simulink model "softMBD"  (R2025b)
settings: Solver=FixedStepAuto  StartTime=0.0  StopTime=30  FixedStep=0.005  RelTol=1e-3
values from neighbouring files (symbols this model uses):
  FPV_mass = 0.8    [Soft.m]
  g = 9.81    [Soft.m]
  ks = 0    [Soft.m]
  p_0 = 1013.25    [Soft.m]
  Q2Ts = forcetomotors()    [Soft.m]    (also in forcetomotors.m = inv(Ts2Q))
  takeOffDuration = 2    [Soft.m]
  Ts = 0.005    [Soft.m]
undefined symbols (not defined in the file or in its folder): CdA, DiscIntNeverNeededParam, kd_pq, kd_pr, kd_y, ki_pq, ki_pr, ki_y, kp_pq, kp_pr, kp_y, pInitialization, rho
libraries: simulink x37, discretizing x11, slpidlib x2, SignalEditorBlockLib x1, simulink_extras x1, shared6dof x1, dynamicsLibrary x1, aerolibasang x1, aerolibnav x1
(part 1 of 20)
settings Model: Creator=rafal  LastModifiedBy=rafal
settings DataIOCC: ReturnWorkspaceOutputs=off
settings OptimizationCC: DefaultParameterBehavior=Inlined  UseDivisionForNetSlopeComputation=on  GainParamInheritBuiltInType=on  UseFloatMulNetSlope=on  InlineInvariantSignals=on  PassReuseOutputArgsAs=Individual arguments  ZeroExternalMemoryAtStartup=off  ZeroInternalMemoryAtStartup=off  NoFixptDivByZeroProtection=on  EfficientFloat2IntCast=on  LifeSpan=1  OptimizeBlockOrder=speed  DifferentSizesBufferReuse=on  EfficientTunableParamExpr=on
settings DebuggingCC: ParameterTunabilityLossMsg=error  BusObjectLabelMismatch=error
settings HardwareCC: ProdBitPerPointer=32.0  ProdBitPerSizeT=32.0  ProdBitPerPtrDiffT=32.0  ProdLargestAtomicInteger=Long  ProdLargestAtomicFloat=Double  ProdWordSize=32.0  ProdLongLongMode=on  ProdHWDeviceType=ARM Compatible->ARM Cortex-M
settings SFSimCC: MATLABDynamicMemAlloc=off
settings RTWCC: SystemTargetFile=ert.tlc  GenCodeOnly=on  TemplateMakefile=ert_default_tmf  Description=Embedded Coder
settings CodeAppCC: ForceParamTrailComments=on  IgnoreCustomStorageClasses=off  OperatorAnnotations=on  SimulinkDataObjDesc=on  SFDataObjDesc=on  CustomSymbolStrGlobalVar=rt$N$M  CustomSymbolStrType=$N$M  CustomSymbolStrFcn=$N$M$F  CustomSymbolStrMacro=$N$M  InsertBlockDesc=on
settings ERTTargetCC: ERTCustomFileTemplate=example_file_process.tlc  ERTFilePackagingFormat=CompactWithDataFile  TargetLangStandard=C99 (ISO)  IncludeMdlTerminateFcn=off  CombineSignalStateStructs=on  SupportContinuousTime=on  SupportNonInlinedSFcns=on

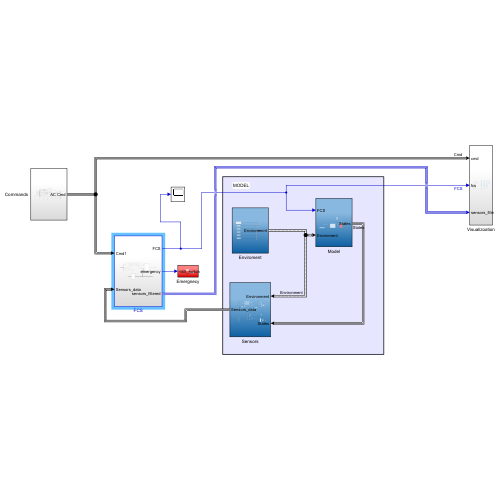
[thumbnail: Simulink's stored preview of the top-level diagram]
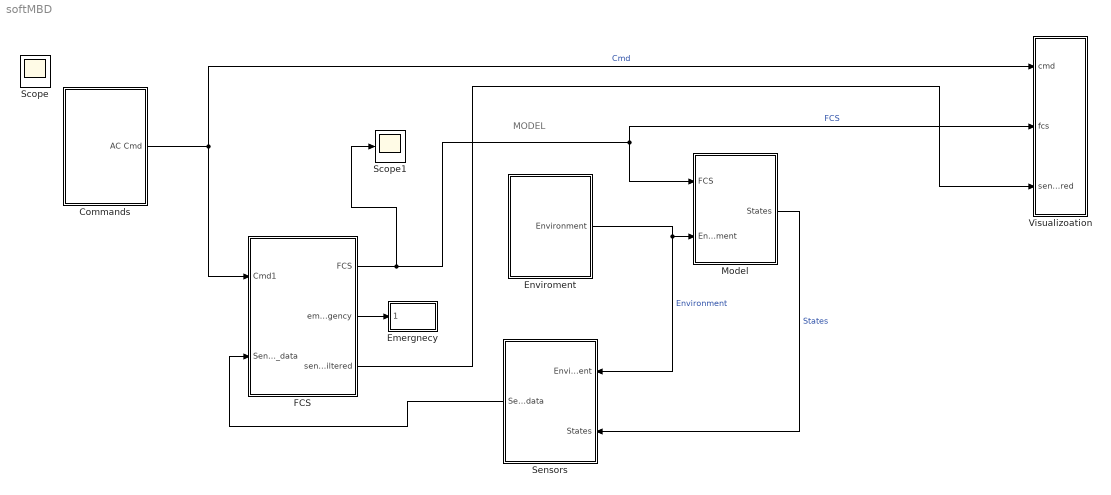
== system softMBD ==
  note: MODEL
  Commands : Subsystem
  Emergnecy : Subsystem
  Enviroment : Subsystem
  FCS : Subsystem
  Model : Subsystem
  Scope1 : Scope
      settings: ActiveDisplayYMinimum=-145.65311813354487  ActiveDisplayYMaximum=2290.6281242370605
  Sensors : Subsystem
  Visualizoation : Subsystem
  Scope : Scope
  wires:
  Model/1(States) -> Sensors/2(States)  "States"
  Sensors/1(Sensors_data) -> FCS/2(Sensors_data)
  Commands/1(AC Cmd) -> Visualizoation/1(cmd), FCS/1(Cmd1)  "Cmd"
  FCS/1(FCS) -> Scope1/1, Visualizoation/2(fcs), Model/1(FCS)  "FCS"
  FCS/2(emergency) -> Emergnecy/1(<kill_switch>)
  Enviroment/1(Environment) -> Sensors/1(Environment), Model/2(Enviroment)  "Environment"
  FCS/3(sensors_filtered) -> Visualizoation/3(sensors_filtered)

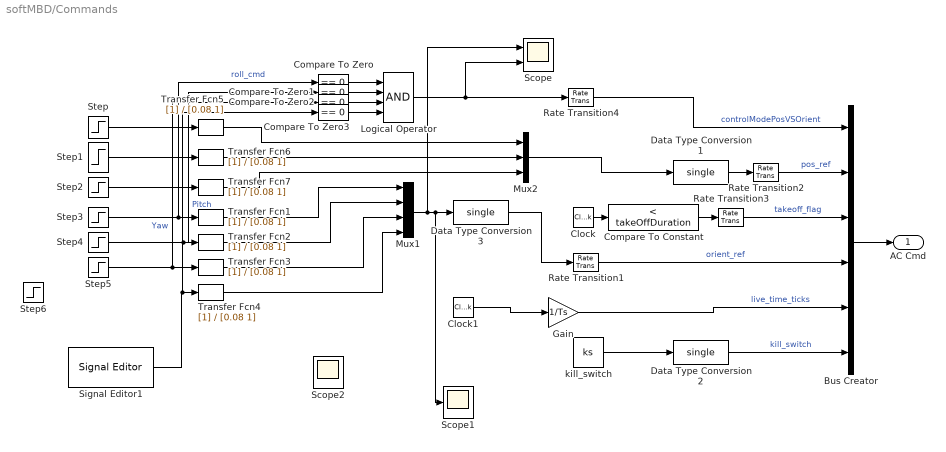
== system softMBD/Commands ==
  Bus Creator : BusCreator  Inputs=6  OutDataTypeStr=Bus: CommandBus
  Clock : DigitalClock  SampleTime=0.005
  Clock1 : DigitalClock  SampleTime=0.005
  Compare To Constant : simulink/Logic and Bit Operations/Compare To Constant  relop=<  const=takeOffDuration  OutDataTypeStr=boolean
  Compare To Zero : simulink/Logic and Bit Operations/Compare To Zero  relop===  OutDataTypeStr=uint8
  Compare To Zero1 : simulink/Logic and Bit Operations/Compare To Zero  relop===  OutDataTypeStr=uint8
  Compare To Zero2 : simulink/Logic and Bit Operations/Compare To Zero  relop===  OutDataTypeStr=boolean
  Compare To Zero3 : simulink/Logic and Bit Operations/Compare To Zero  relop===  OutDataTypeStr=boolean
  Data Type Conversion1 : DataTypeConversion  OutDataTypeStr=single  SaturateOnIntegerOverflow=off  RndMeth=Floor
  Data Type Conversion2 : DataTypeConversion  OutDataTypeStr=single  SaturateOnIntegerOverflow=off  RndMeth=Floor
  Data Type Conversion3 : DataTypeConversion  OutDataTypeStr=single  SaturateOnIntegerOverflow=off  RndMeth=Floor
  Gain : Gain  Gain=1/Ts  OutDataTypeStr=single
  Logical Operator : Logic  Inputs=4  AllPortsSameDT=off  OutDataTypeStr=boolean
  Mux1 : Mux
  Mux2 : Mux  Inputs=3
  Rate Transition{1..4} (4 alike) : RateTransition  OutPortSampleTime=Ts
  Scope : Scope  NumInputPorts=2
      settings: ActiveDisplayYMinimum=-0.12499999999999997  ActiveDisplayYMaximum=1.125  DataLoggingVariableName=ScopeData74
  Scope1 : Scope
      settings: ActiveDisplayYMinimum=-1  ActiveDisplayYMaximum=1  DataLoggingVariableName=ScopeData25
  Scope2 : Scope
      settings: ActiveDisplayYMinimum=-0.11809653934888488  ActiveDisplayYMaximum=1.0178996154832094  DataLoggingVariableName=ScopeData40
  Signal Editor1 : SignalEditorBlockLib/Signal Editor  FileName=signal-test.mat  ActiveScenario=Scenario  ActiveSignal=Signal 1  IsBus=off  OutputBusObjectStr=Bus: BusObject  SampleTime=0  ZeroCross=off  OutputAfterFinalValue=Setting to zero  Unit=inherit  PreserveSignalName=on  ApplySigPropsToAllScenarios=on  ApplySigPropsToAllSignals=off  SignalPropertySource=Dialog parameters
  Step{,1..5} (6 alike) : Step  After=0  SampleTime=0
  Step6 : Step  Time=2  Before=1  After=0  SampleTime=0
  Transfer Fcn{1..7} (7 alike) : TransferFcn  Denominator=[0.08 1]
  kill_switch : Constant  Value=ks
  AC Cmd : Outport  OutDataTypeStr=Bus: CommandBus  VectorParamsAs1DForOutWhenUnconnected=off
  wires:
  Rate Transition4/1 -> Bus Creator/1  "controlModePosVSOrient"
  Gain/1 -> Bus Creator/5  "live_time_ticks"
  Clock/1 -> Compare To Constant/1
  Step1/1 -> Transfer Fcn6/1
  Rate Transition2/1 -> Bus Creator/2  "pos_ref"
  Step2/1 -> Transfer Fcn7/1
  Mux1/1 -> Scope/1, Scope1/1, Data Type Conversion3/1
  Bus Creator/1 -> AC Cmd/1
  Compare To Constant/1 -> Rate Transition3/1
  Step4/1 -> Compare To Zero1/1, Transfer Fcn2/1  "Pitch"
  Data Type Conversion1/1 -> Rate Transition2/1
  Data Type Conversion3/1 -> Rate Transition1/1
  Step/1 -> Transfer Fcn5/1
  Mux2/1 -> Data Type Conversion1/1
  Rate Transition1/1 -> Bus Creator/4  "orient_ref"
  Step5/1 -> Compare To Zero2/1, Transfer Fcn3/1  "Yaw"
  Rate Transition3/1 -> Bus Creator/3  "takeoff_flag"
  Compare To Zero/1 -> Logical Operator/1
  Compare To Zero1/1 -> Logical Operator/2
  Compare To Zero2/1 -> Logical Operator/3
  kill_switch/1 -> Data Type Conversion2/1
  Data Type Conversion2/1 -> Bus Creator/6  "kill_switch"
  Clock1/1 -> Gain/1
  Step3/1 -> Compare To Zero/1, Transfer Fcn1/1  "roll_cmd"
  Transfer Fcn1/1 -> Mux1/1
  Transfer Fcn3/1 -> Mux1/3
  Transfer Fcn4/1 -> Mux1/4
  Transfer Fcn5/1 -> Mux2/1
  Transfer Fcn6/1 -> Mux2/2
  Transfer Fcn7/1 -> Mux2/3
  Compare To Zero3/1 -> Logical Operator/4
  Transfer Fcn2/1 -> Mux1/2
  Logical Operator/1 -> Rate Transition4/1, Scope/2
  Signal Editor1/1 -> Compare To Zero3/1, Transfer Fcn4/1

== system softMBD/Emergnecy ==
  <kill_switch> : Inport
  If : If
  Switch Case Action Subsystem : Subsystem  TreatAsAtomicUnit=on
  Terminator : Terminator
  Zero : Constant  OutDataTypeStr=Inherit: Inherit via back propagation
  wires:
  If/1 -> Switch Case Action Subsystem/Action
  If/2 -> Terminator/1
  Switch Case Action Subsystem/1(emergency) -> ?
  Zero/1 -> Switch Case Action Subsystem/1(In1)
  <kill_switch>/1 -> If/1

== system softMBD/Enviroment ==
  Air Density : Constant  Value=1.225  OutDataTypeStr=single
  Air Temp : Constant  Value=288  OutDataTypeStr=single
  Bus Creator : BusCreator  Inputs=6  OutDataTypeStr=Bus: AtmosphereBus  NonVirtualBus=on
  Gravity : Constant  Value=[0 0 9.81]  OutDataTypeStr=single
  Magnetic Field : Constant  Value=[0 0 0]  OutDataTypeStr=single
  Pressure : Constant  Value=1013.25  OutDataTypeStr=single
  Speed of Sound : Constant  Value=340  OutDataTypeStr=single
  Environment : Outport  VectorParamsAs1DForOutWhenUnconnected=off
  wires:
  Magnetic Field/1 -> Bus Creator/6  "MagneticField_ned"
  Air Density/1 -> Bus Creator/5  "air_density"
  Air Temp/1 -> Bus Creator/2  "air_temp"
  Gravity/1 -> Bus Creator/1  "Gravity_ned"
  Speed of Sound/1 -> Bus Creator/3  "speed_sound"
  Bus Creator/1 -> Environment/1
  Pressure/1 -> Bus Creator/4  "pressure"

== system softMBD/FCS ==
  Cmd1 : Inport
  Sensors_data : Inport  Port=2
  Bus Selector : BusSelector  OutputSignals=controlModePosVSOrient,orient_ref,takeoff_flag,pos_ref,kill_switch
  Controller : Subsystem
  filters : Subsystem
  value scaling : Subsystem
  FCS : Outport
  emergency : Outport  Port=2
  sensors_filtered : Outport  Port=3
  wires:
  Cmd1/1 -> Bus Selector/1
  Controller/1(FCS) -> FCS/1
  Bus Selector/1 -> Controller/1(In1)  "<controlModePosVSOrient>"
  Bus Selector/3 -> Controller/3(In3)  "<takeoff_flag>"
  Bus Selector/4 -> Controller/4(In4)  "<pos_ref>"
  Sensors_data/1 -> filters/1(Sensors_data)
  filters/1(Sensors_filtered) -> sensors_filtered/1, Controller/5(Sensors_filtered)  "sensors_filtered"
  Bus Selector/5 -> emergency/1  "<kill_switch>"
  Bus Selector/2 -> value scaling/1(<orient_ref>)  "<orient_ref>"
  value scaling/1(Out1) -> Controller/2(In2)

== system softMBD/Model ==
  FCS : Inport
  Enviroment : Inport  Port=2
  6DOF (Quaternion)1 : shared6dof/6DOF (Euler Angles)  units=Metric (MKS)  mtype=Fixed  rep=Euler Angles  xme_0=[0 0 0]  Vm_0=[0 0 0]  eul_0=[0 0 0]  pm_0=[0 0 0]  mass_0=FPV_mass  mass_e=0.5  mass_f=2.0  inertia=diag([0.003, 0.003, 0.005])  inertia_e=eye(3)  inertia_f=2*eye(3)  k_quat=Vehicle.SixDOF.quatGain  vre_flag=on  abi_flag=on  aMode=aMode  xme_statename=''  Vm_statename=''  eul_statename=''  quat_statename=''  pm_statename=''  mass_statename=''
  Abs : Abs  SaturateOnIntegerOverflow=off
  Add : Sum  Inputs=+++
  Bias : Bias  Bias=-48  SaturateOnIntegerOverflow=off
  Bias1 : Bias  Bias=200  SaturateOnIntegerOverflow=off
  Bus Creator : BusCreator  Inputs=8
  Bus Selector : BusSelector  OutputSignals=air_density
  Constant : Constant  Value=630*[1 1 1 1]  VectorParams1D=off
  Constant2 : Constant  Value=FPV_mass*g*[0 0 1]
  Data Type Conversion2 : DataTypeConversion  OutDataTypeStr=double  SaturateOnIntegerOverflow=off  RndMeth=Floor
  Data Type Conversion3 : DataTypeConversion  OutDataTypeStr=double  SaturateOnIntegerOverflow=off  RndMeth=Floor
  Gain : Gain  Commented=on  Gain=[1; 1; -1]
  Gain1 : Gain  Gain=(4184-200)/1999
  Gain2 : Gain  Gain=[1 -1 -1 1]
  Gain3 : Gain  Gain=-1/2*rho*CdA
  Matrix Multiply : Product  Multiplication=Matrix(*)
  Multirotor : Multirotor  armLength=0.11  radius=0.0635
  Product : Product
  Saturation : Saturate  UpperLimit=4184  LowerLimit=200
  Scope1 : Scope  NumInputPorts=3
      settings: ActiveDisplayYMinimum=-17.244801664132787  ActiveDisplayYMaximum=11.437507576273727  DataLoggingVariableName=ScopeData54
  Scope2 : Scope  NumInputPorts=2
      settings: ActiveDisplayYMinimum=-2865.3748027143724  ActiveDisplayYMaximum=2716.5327218117013  DataLoggingVariableName=ScopeData62
  Scope3 : Scope  NumInputPorts=4
      settings: ActiveDisplayYMinimum=-27.905959147776141  ActiveDisplayYMaximum=16.159289367560238  DataLoggingVariableName=ScopeData64
  Scope4 : Scope  NumInputPorts=2
      settings: ActiveDisplayYMinimum=-1  ActiveDisplayYMaximum=1  DataLoggingVariableName=ScopeData38
  Subsystem : Subsystem  Commented=on
  Terminator : Terminator
  States : Outport
  wires:
  6DOF (Quaternion)1/1 -> Scope3/1, Bus Creator/1  "V_e"
  6DOF (Quaternion)1/2 -> Scope3/4, Bus Creator/2  "x_e"
  6DOF (Quaternion)1/3 -> Bus Creator/3  "Euler"
  Bus Creator/1 -> States/1
  6DOF (Quaternion)1/4 -> Bus Creator/4  "DCM_be"
  6DOF (Quaternion)1/5 -> Abs/1, Bus Creator/5, Gain3/1  "V_b"
  6DOF (Quaternion)1/6 -> Scope3/3, Bus Creator/6  "omega_b"
  6DOF (Quaternion)1/7 -> Bus Creator/7  "Domega_b"
  6DOF (Quaternion)1/8 -> Scope3/2, Bus Creator/8  "Accel_b"
  Subsystem/1(F_xyz) -> Gain/1
  Bias/1 -> Gain1/1
  Saturation/1 -> Gain2/1
  Constant2/1 -> Add/2
  Enviroment/1 -> Bus Selector/1
  Data Type Conversion2/1 -> Multirotor/2
  Multirotor/1 -> Scope1/1, Add/3
  Bias1/1 -> Saturation/1
  Multirotor/2 -> Scope4/1, 6DOF (Quaternion)1/2
  FCS/1 -> Scope2/1, Data Type Conversion3/1
  Bus Selector/1 -> Data Type Conversion2/1  "<air_density>"
  Gain1/1 -> Bias1/1
  Data Type Conversion3/1 -> Bias/1
  Add/1 -> 6DOF (Quaternion)1/1, Scope1/2
  6DOF (Quaternion)1/9 -> Terminator/1  "Accel_b"
  Gain2/1 -> Scope2/2, Multirotor/1
  Gain3/1 -> Product/2
  Abs/1 -> Product/1
  Product/1 -> Add/1, Scope1/3

== system softMBD/Sensors ==
  note: altitude_sonar
  Environment : Inport
  States : Inport  Port=2
  Assumes takeoff was level1 : Bias  Commented=on  Bias=p_0  SaturateOnIntegerOverflow=off
  Bus Selector : BusSelector  Commented=on  OutputSignals=Accel_b,omega_b,Domega_b,DCM_be,x_e
  Bus Selector1 : BusSelector  Commented=on  OutputSignals=Gravity_ned
  Bus Selector2 : BusSelector  OutputSignals=x_e,V_e,omega_b,Accel_b
  CG location : Constant  Commented=on  Value=[0 0 0]
  Data Type Conversion1 : DataTypeConversion  Commented=on  OutDataTypeStr=single  SaturateOnIntegerOverflow=off  RndMeth=Floor
  Data Type Conversion2 : DataTypeConversion  Commented=on  OutDataTypeStr=single  SaturateOnIntegerOverflow=off  RndMeth=Floor
  Data Type Conversion3 : DataTypeConversion  Commented=on  OutDataTypeStr=single  SaturateOnIntegerOverflow=off  RndMeth=Floor
  Demux : Demux  Commented=on  Outputs=3
  Demux1 : Demux  Commented=on  Outputs=3
  Demux2 : Demux  Outputs=3
  Demux3 : Demux  Outputs=3
  Matrix Multiply : Product  Commented=on  Multiplication=Matrix(*)
  Memory : Memory  Commented=on
  Mux : Mux  Commented=on  Inputs=8
  Mux2 : Mux  Inputs=3
  Rate Transition : RateTransition  Commented=on
  Rate Transition1 : RateTransition
  Saturation : Saturate  Commented=on  UpperLimit=inf  LowerLimit=0  OutDataTypeStr=single
  Scope : Scope  Commented=on  NumInputPorts=3
      settings: ActiveDisplayYMinimum=-74.251567840576172  ActiveDisplayYMaximum=64.477069854736328  DataLoggingVariableName=ScopeData44
  Scope1 : Scope  Commented=on  NumInputPorts=3
      settings: ActiveDisplayYMinimum=-0.22507907450199127  ActiveDisplayYMaximum=0.16993089020252228  DataLoggingVariableName=ScopeData48
  Scope2 : Scope  Commented=on
      settings: ActiveDisplayYMinimum=-1  ActiveDisplayYMaximum=1  DataLoggingVariableName=ScopeData65
  Scope3 : Scope
      settings: ActiveDisplayYMinimum=-1  ActiveDisplayYMaximum=1  DataLoggingVariableName=ScopeData63
  Selector : Selector  Commented=on  InputPortWidth=3  IndexOptions=Index vector (dialog)  Indices=[3]  OutputSizes=1
  Subsystem : Subsystem  Commented=on
  Subsystem1 : Subsystem
  Terminator1 : Terminator
  Terminator2 : Terminator
  Terminator3 : Terminator
  Three-axis Inertial Measurement Unit1 : aerolibnav/Three-axis Inertial Measurement Unit  Commented=on  units=Metric (MKS)  imu=[0 0 0]  i_Ts=0  dtype_a=on  w_a=190  z_a=0.707  a_sf_cc=[1 0 0; 0 1 0; 0 0 1]  a_bias=[0 0 0]  a_sat="[-inf  -inf  -inf  inf inf inf]"  dtype_g=on  w_g=190  z_g=0.707  g_sf_cc=[1 0 0; 0 1 0; 0 0 1]  g_bias=[0 0 0]  g_sens=[0 0 0]  g_sat="[-inf  -inf  -inf  inf inf inf]"  i_rand=on  i_seeds=[23093 23094 23095 23096 23097 23098]  i_pow=[0.001 0.001 0.001 0.0001 0.0001 0.0001]
  altToprs_gain : Gain  Commented=on  Gain=12.017  ParamDataTypeStr=single  OutDataTypeStr=single
  altToprs_gain1 : Gain  Commented=on  Gain=-1  ParamDataTypeStr=single  OutDataTypeStr=double
  altToprs_gain2 : Gain  Gain=-1  ParamDataTypeStr=single  OutDataTypeStr=double
  altToprs_gain3 : Gain  Gain=-1  ParamDataTypeStr=single  OutDataTypeStr=double
  Sensors_data : Outport
  wires:
  Memory/1 -> Bus Selector/1
  Environment/1 -> Bus Selector1/1
  Bus Selector1/1 -> Matrix Multiply/2  "<Gravity_ned>"
  Bus Selector/4 -> Matrix Multiply/1  "<DCM_be>"
  CG location/1 -> Three-axis Inertial Measurement Unit1/4
  Matrix Multiply/1 -> Scope2/1, Three-axis Inertial Measurement Unit1/5
  Bus Selector/5 -> Selector/1  "<x_e>"
  Bus Selector/3 -> Three-axis Inertial Measurement Unit1/3  "<Domega_b>"
  Bus Selector/2 -> Three-axis Inertial Measurement Unit1/2  "<omega_b>"
  Bus Selector/1 -> Three-axis Inertial Measurement Unit1/1  "<Accel_b>"
  Selector/1 -> altToprs_gain/1, altToprs_gain1/1
  Saturation/1 -> Mux/8  "prs"
  Demux/1 -> Mux/1, Scope/1  "ddx"
  Demux/2 -> Mux/2, Scope/2  "ddy"
  Demux/3 -> Mux/3, Scope/3  "ddz"
  Demux1/1 -> Scope1/1, Mux/4  "p"
  Demux1/2 -> Scope1/2, Mux/5  "q"
  Demux1/3 -> Scope1/3, Mux/6  "r"
  Subsystem/1(Out1) -> Rate Transition/1
  altToprs_gain1/1 -> Saturation/1
  altToprs_gain/1 -> Assumes takeoff was level1/1
  Assumes takeoff was level1/1 -> Data Type Conversion2/1
  Three-axis Inertial Measurement Unit1/1 -> Data Type Conversion3/1  "prs"
  Data Type Conversion3/1 -> Demux/1
  Three-axis Inertial Measurement Unit1/2 -> Data Type Conversion1/1  "prs"
  Data Type Conversion1/1 -> Demux1/1
  Data Type Conversion2/1 -> Mux/7
  Demux2/3 -> altToprs_gain2/1
  Demux3/2 -> Mux2/2
  Rate Transition1/1 -> Sensors_data/1
  Demux3/1 -> Mux2/1
  Demux2/2 -> Terminator1/1
  Bus Selector2/1 -> Demux2/1  "<x_e>"
  altToprs_gain2/1 -> Scope3/1, Subsystem1/1(In1)
  Demux3/3 -> altToprs_gain3/1
  altToprs_gain3/1 -> Mux2/3
  States/1 -> Bus Selector2/1
  Mux2/1 -> Terminator3/1
  Subsystem1/1(Out1) -> Rate Transition1/1
  Demux2/1 -> Terminator2/1
  Bus Selector2/2 -> Demux3/1  "<V_e>"
  Bus Selector2/3 -> Subsystem1/2(In2)  "<omega_b>"
  Bus Selector2/4 -> Subsystem1/3(<Accel_b>)  "<Accel_b>"
  Mux/1 -> Subsystem/1(In1)

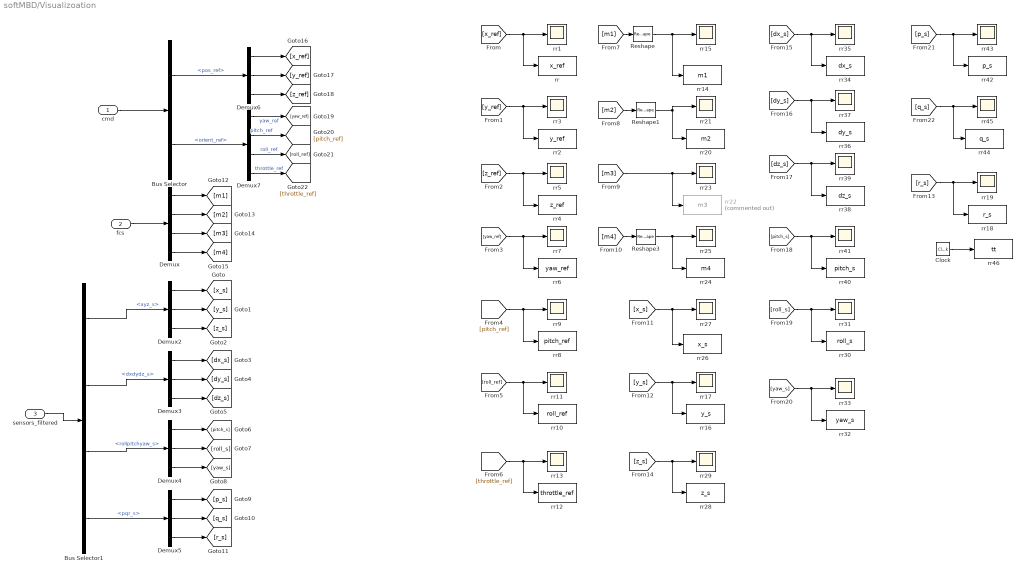
== system softMBD/Visualizoation ==
  cmd : Inport
  fcs : Inport  Port=2
  sensors_filtered : Inport  Port=3
  Bus Selector : BusSelector  OutputSignals=pos_ref,orient_ref
  Bus Selector1 : BusSelector  OutputSignals=xyz_s,dxdydz_s,rollpitchyaw_s,pqr_s
  Clock : DigitalClock  SampleTime=0.005
  Demux : Demux
  Demux{2..6} (5 alike) : Demux  Outputs=3
  Demux7 : Demux
  Reshape : Reshape
  Reshape1 : Reshape
  Reshape3 : Reshape
  rr : ToWorkspace  VariableName=x_ref  SampleTime=Ts
  rr{1,3,5,7,9,11,13,15,17,19,21,23,25,27,29,31,33,35,37,39,41,43,45} (23 alike) : Scope
      rr1 settings: ActiveDisplayYMinimum=-1  ActiveDisplayYMaximum=1  DataLoggingVariableName=ScopeData10
      rr11 settings: ActiveDisplayYMinimum=-1  ActiveDisplayYMaximum=1  DataLoggingVariableName=ScopeData6
      rr13 settings: ActiveDisplayYMinimum=-1  ActiveDisplayYMaximum=1  DataLoggingVariableName=ScopeData7
      rr15 settings: ActiveDisplayYMinimum=-73.950467746195855  ActiveDisplayYMaximum=1145.5542097157629  DataLoggingVariableName=ScopeData8
      rr17 settings: ActiveDisplayYMinimum=-1  ActiveDisplayYMaximum=1  DataLoggingVariableName=ScopeData9
      rr19 settings: ActiveDisplayYMinimum=-1  ActiveDisplayYMaximum=1  DataLoggingVariableName=ScopeData11
      rr21 settings: ActiveDisplayYMinimum=38  ActiveDisplayYMaximum=58  DataLoggingVariableName=ScopeData12
      rr23 settings: ActiveDisplayYMinimum=-70.597177763307627  ActiveDisplayYMaximum=1115.3745998697689  DataLoggingVariableName=ScopeData13
      rr25 settings: ActiveDisplayYMinimum=46.949385488802776  ActiveDisplayYMaximum=57.45553060077502  DataLoggingVariableName=ScopeData14
      rr27 settings: ActiveDisplayYMinimum=-1  ActiveDisplayYMaximum=1  DataLoggingVariableName=ScopeData15
      rr29 settings: ActiveDisplayYMinimum=-248.57406984307249  ActiveDisplayYMaximum=124.72069577188705  DataLoggingVariableName=ScopeData16
      rr3 settings: ActiveDisplayYMinimum=-5  ActiveDisplayYMaximum=5  DataLoggingVariableName=ScopeData2
      rr31 settings: ActiveDisplayYMinimum=-1  ActiveDisplayYMaximum=1  DataLoggingVariableName=ScopeData17
      rr33 settings: ActiveDisplayYMinimum=-1  ActiveDisplayYMaximum=1  DataLoggingVariableName=ScopeData18
      rr35 settings: ActiveDisplayYMinimum=-1  ActiveDisplayYMaximum=1  DataLoggingVariableName=ScopeData19
      rr37 settings: ActiveDisplayYMinimum=-1  ActiveDisplayYMaximum=1  DataLoggingVariableName=ScopeData20
      rr39 settings: ActiveDisplayYMinimum=-1  ActiveDisplayYMaximum=1  DataLoggingVariableName=ScopeData21
      rr41 settings: ActiveDisplayYMinimum=-1  ActiveDisplayYMaximum=1  DataLoggingVariableName=ScopeData22
      rr43 settings: ActiveDisplayYMinimum=-1  ActiveDisplayYMaximum=1  DataLoggingVariableName=ScopeData23
      rr45 settings: ActiveDisplayYMinimum=-1  ActiveDisplayYMaximum=1  DataLoggingVariableName=ScopeData24
      rr5 settings: ActiveDisplayYMinimum=-1  ActiveDisplayYMaximum=1  DataLoggingVariableName=ScopeData3
      rr7 settings: ActiveDisplayYMinimum=-5  ActiveDisplayYMaximum=5  DataLoggingVariableName=ScopeData4
      rr9 settings: ActiveDisplayYMinimum=-5  ActiveDisplayYMaximum=5  DataLoggingVariableName=ScopeData5
  rr10 : ToWorkspace  VariableName=roll_ref  SampleTime=Ts
  rr12 : ToWorkspace  VariableName=throttle_ref  SampleTime=Ts
  rr14 : ToWorkspace  VariableName=m1  SampleTime=Ts
  rr16 : ToWorkspace  VariableName=y_s  SampleTime=Ts
  rr18 : ToWorkspace  VariableName=r_s  SampleTime=Ts
  rr2 : ToWorkspace  VariableName=y_ref  SampleTime=Ts
  rr20 : ToWorkspace  VariableName=m2  SampleTime=Ts
  rr22 : ToWorkspace  Commented=on  VariableName=m3  SampleTime=Ts
  rr24 : ToWorkspace  VariableName=m4  SampleTime=Ts
  rr26 : ToWorkspace  VariableName=x_s  SampleTime=Ts
  rr28 : ToWorkspace  VariableName=z_s  SampleTime=Ts
  rr30 : ToWorkspace  VariableName=roll_s  SampleTime=Ts
  rr32 : ToWorkspace  VariableName=yaw_s  SampleTime=Ts
  rr34 : ToWorkspace  VariableName=dx_s  SampleTime=Ts
  rr36 : ToWorkspace  VariableName=dy_s  SampleTime=Ts
  rr38 : ToWorkspace  VariableName=dz_s  SampleTime=Ts
  rr4 : ToWorkspace  VariableName=z_ref  SampleTime=Ts
  rr40 : ToWorkspace  VariableName=pitch_s  SampleTime=Ts
  rr42 : ToWorkspace  VariableName=p_s  SampleTime=Ts
  rr44 : ToWorkspace  VariableName=q_s  SampleTime=Ts
  rr46 : ToWorkspace  VariableName=tt  SampleTime=Ts
  rr6 : ToWorkspace  VariableName=yaw_ref  SampleTime=Ts
  rr8 : ToWorkspace  VariableName=pitch_ref  SampleTime=Ts
  wires:
  cmd/1 -> Bus Selector/1
  sensors_filtered/1 -> Bus Selector1/1
  fcs/1 -> Demux/1
  Demux2/3 -> [z_s]
  Demux2/2 -> [y_s]
  Demux2/1 -> [x_s]
  Demux3/3 -> [dz_s]
  Demux3/2 -> [dy_s]
  Demux3/1 -> [dx_s]
  Demux4/3 -> [yaw_s]
  Demux4/2 -> [roll_s]
  Demux4/1 -> [pitch_s]
  Demux5/3 -> [r_s]
  Demux5/2 -> [q_s]
  Demux5/1 -> [p_s]
  Demux/1 -> [m1]
  Demux/4 -> [m4]
  Demux/3 -> [m3]
  Demux/2 -> [m2]
  Demux6/1 -> [x_ref]
  Bus Selector/2 -> Demux7/1  "<orient_ref>"
  Demux7/1 -> [yaw_ref]  "yaw_ref"
  Demux6/3 -> [z_ref]
  Demux7/2 -> [pitch_ref]  "pitch_ref"
  Demux7/3 -> [roll_ref]  "roll_ref"
  Demux6/2 -> [y_ref]
  Bus Selector/1 -> Demux6/1  "<pos_ref>"
  [x_ref] -> rr/1, rr1/1
  Demux7/4 -> [throttle_ref]  "throttle_ref"
  [y_ref] -> rr2/1, rr3/1
  [z_ref] -> rr4/1, rr5/1
  [yaw_ref] -> rr6/1, rr7/1
  [pitch_ref] -> rr8/1, rr9/1
  [roll_ref] -> rr10/1, rr11/1
  [throttle_ref] -> rr12/1, rr13/1
  [y_s] -> rr16/1, rr17/1
  [x_s] -> rr26/1, rr27/1
  [m1] -> Reshape/1
  [m4] -> Reshape3/1
  [r_s] -> rr18/1, rr19/1
  [roll_s] -> rr30/1, rr31/1
  [dx_s] -> rr34/1, rr35/1
  [dy_s] -> rr36/1, rr37/1
  [pitch_s] -> rr40/1, rr41/1
  [z_s] -> rr28/1, rr29/1
  [dz_s] -> rr38/1, rr39/1
  [yaw_s] -> rr32/1, rr33/1
  [p_s] -> rr42/1, rr43/1
  [q_s] -> rr44/1, rr45/1
  Bus Selector1/1 -> Demux2/1  "<xyz_s>"
  Bus Selector1/2 -> Demux3/1  "<dxdydz_s>"
  Bus Selector1/3 -> Demux4/1  "<rollpitchyaw_s>"
  Bus Selector1/4 -> Demux5/1  "<pqr_s>"
  Clock/1 -> rr46/1
  Reshape/1 -> rr14/1, rr15/1
  [m2] -> Reshape1/1
  [m3] -> rr22/1, rr23/1
  Reshape3/1 -> rr24/1, rr25/1
  Reshape1/1 -> rr21/1, rr20/1

== system softMBD/Emergnecy/Switch Case Action Subsystem ==
  In1 : Inport
  Action Port : ActionPort  ActionPortLabel=if(u1 > 0)
  emergency : Outport
  wires:
  In1/1 -> emergency/1

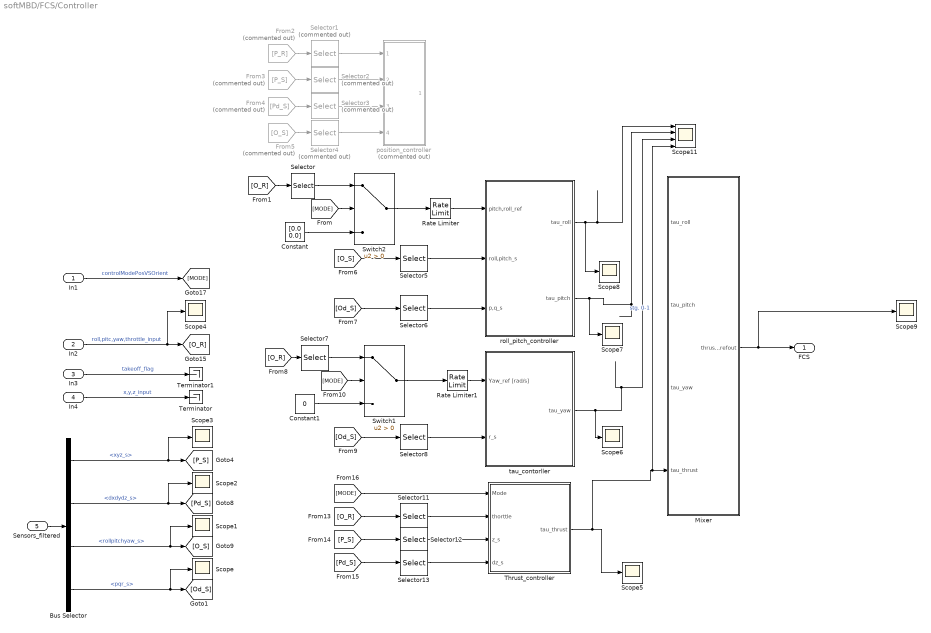
== system softMBD/FCS/Controller ==
  In1 : Inport
  In2 : Inport  Port=2
  In3 : Inport  Port=3
  In4 : Inport  Port=4
  Sensors_filtered : Inport  Port=5
  Bus Selector : BusSelector  OutputSignals=xyz_s,dxdydz_s,rollpitchyaw_s,pqr_s
  Constant : Constant  Value=[0.0 0.0]
  Constant1 : Constant  Value=0
  From2 : From  Commented=on  GotoTag=P_R
  From3 : From  Commented=on  GotoTag=P_S
  From4 : From  Commented=on  GotoTag=Pd_S
  From5 : From  Commented=on  GotoTag=O_S
  Mixer : Subsystem
  Rate Limiter : RateLimiter  RisingSlewLimit=3.0  FallingSlewLimit=-3.0  SampleTimeMode=inherited
  Rate Limiter1 : RateLimiter  RisingSlewLimit=20  FallingSlewLimit=-20  SampleTimeMode=inherited
  Scope{,1..9} (10 alike) : Scope
      Scope settings: ActiveDisplayYMinimum=-1  ActiveDisplayYMaximum=1  DataLoggingVariableName=ScopeData26
      Scope1 settings: ActiveDisplayYMinimum=-1  ActiveDisplayYMaximum=1  DataLoggingVariableName=ScopeData27
      Scope2 settings: ActiveDisplayYMinimum=-1  ActiveDisplayYMaximum=1  DataLoggingVariableName=ScopeData28
      Scope3 settings: ActiveDisplayYMinimum=-198.01537047970481  ActiveDisplayYMaximum=949.36258849660373  DataLoggingVariableName=ScopeData29
      Scope4 settings: ActiveDisplayYMinimum=-0.61312502622604359  ActiveDisplayYMaximum=5.5181252360343933  DataLoggingVariableName=ScopeData30
      Scope5 settings: ActiveDisplayYMinimum=-1.734030298247256  ActiveDisplayYMaximum=15.492532201752745  DataLoggingVariableName=ScopeData31
      Scope6 settings: ActiveDisplayYMinimum=-1  ActiveDisplayYMaximum=1  DataLoggingVariableName=ScopeData32
      Scope7 settings: ActiveDisplayYMinimum=-1  ActiveDisplayYMaximum=1  DataLoggingVariableName=ScopeData33
      Scope8 settings: ActiveDisplayYMinimum=-0.39374999329447746  ActiveDisplayYMaximum=0.043749999254941933  DataLoggingVariableName=ScopeData34
      Scope9 settings: ActiveDisplayYMinimum=-1.4489088058471395  ActiveDisplayYMaximum=1200.2335538864136  DataLoggingVariableName=ScopeData35
  Scope11 : Scope  NumInputPorts=4
      settings: ActiveDisplayYMinimum=-1.7687499932944772  ActiveDisplayYMaximum=12.418749999254942  DataLoggingVariableName=ScopeData66
  Selector : Selector  InputPortWidth=4  IndexOptions=Index vector (dialog)  Indices=[1 2]  OutputSizes=1
  Selector1 : Selector  Commented=on  InputPortWidth=3  IndexOptions=Index vector (dialog)  Indices=[1 2]  OutputSizes=1
  Selector11 : Selector  InputPortWidth=4  IndexOptions=Index vector (dialog)  Indices=[4]  OutputSizes=1
  Selector12 : Selector  InputPortWidth=3  IndexOptions=Index vector (dialog)  Indices=[3]  OutputSizes=1
  Selector13 : Selector  InputPortWidth=3  IndexOptions=Index vector (dialog)  Indices=[3]  OutputSizes=1
  Selector2 : Selector  Commented=on  InputPortWidth=3  IndexOptions=Index vector (dialog)  Indices=[1 2]  OutputSizes=1
  Selector3 : Selector  Commented=on  InputPortWidth=3  IndexOptions=Index vector (dialog)  Indices=[1 2]  OutputSizes=1
  Selector4 : Selector  Commented=on  InputPortWidth=3  IndexOptions=Index vector (dialog)  Indices=[3]  OutputSizes=1
  Selector5 : Selector  InputPortWidth=3  IndexOptions=Index vector (dialog)  Indices=[1 2]  OutputSizes=1
  Selector6 : Selector  InputPortWidth=3  IndexOptions=Index vector (dialog)  Indices=[1 2]  OutputSizes=1
  Selector7 : Selector  InputPortWidth=4  IndexOptions=Index vector (dialog)  Indices=[3]  OutputSizes=1
  Selector8 : Selector  InputPortWidth=3  IndexOptions=Index vector (dialog)  Indices=[3]  OutputSizes=1
  Switch1 : Switch  Criteria=u2 > Threshold  OutDataTypeStr=single  SaturateOnIntegerOverflow=off  InputSameDT=off
  Switch2 : Switch  Criteria=u2 > Threshold  OutDataTypeStr=single  SaturateOnIntegerOverflow=off  InputSameDT=off
  Terminator : Terminator
  Terminator1 : Terminator
  Thrust_controller : Subsystem
  position_controller : Subsystem  Commented=on
  roll_pitch_controller : Subsystem
  tau_contorller : Subsystem
  FCS : Outport
  wires:
  Mixer/1(thrusts_refout) -> Scope9/1, FCS/1
  In1/1 -> [MODE]  "controlModePosVSOrient"
  In2/1 -> Scope4/1, [O_R]  "roll,pitc,yaw,throttle_input"
  In3/1 -> Terminator1/1  "takeoff_flag"
  In4/1 -> Terminator/1  "x,y,z_input"
  Sensors_filtered/1 -> Bus Selector/1
  Bus Selector/2 -> Scope2/1, [Pd_S]  "<dxdydz_s>"
  Bus Selector/1 -> Scope3/1, [P_S]  "<xyz_s>"
  roll_pitch_controller/1(tau_roll) -> Scope8/1, Scope11/1
  roll_pitch_controller/2(tau_pitch) -> Scope7/1, Scope11/2
  tau_contorller/1(tau_yaw) -> Scope6/1, Scope11/3
  [MODE] -> Switch2/2
  From2/1 -> Selector1/1
  Selector1/1 -> position_controller/1(x_y_ref)
  Bus Selector/4 -> Scope/1, [Od_S]  "<pqr_s>"
  Bus Selector/3 -> Scope1/1, [O_S]  "<rollpitchyaw_s>"
  From3/1 -> Selector2/1
  From4/1 -> Selector3/1
  Selector2/1 -> position_controller/2(x,y,_s)
  Selector3/1 -> position_controller/3(dx,dy_s)
  From5/1 -> Selector4/1
  Selector4/1 -> position_controller/4(yaw_s)
  [O_S] -> Selector5/1
  [Od_S] -> Selector6/1
  Selector5/1 -> roll_pitch_controller/2(roll,pitch_s)
  Selector6/1 -> roll_pitch_controller/3(p,q_s)
  Selector8/1 -> tau_contorller/2(r_s)
  [Od_S] -> Selector8/1
  [O_R] -> Selector11/1
  Selector11/1 -> Thrust_controller/2(thorttle)
  Selector12/1 -> Thrust_controller/3(z_s)
  Selector13/1 -> Thrust_controller/4(dz_s)
  [P_S] -> Selector12/1
  [Pd_S] -> Selector13/1
  [MODE] -> Thrust_controller/1(Mode)
  Rate Limiter/1 -> roll_pitch_controller/1(pitch,roll_ref)
  [MODE] -> Switch1/2
  Switch1/1 -> Rate Limiter1/1
  Switch2/1 -> Rate Limiter/1
  Rate Limiter1/1 -> tau_contorller/1(Yaw_ref [rad/s])
  Thrust_controller/1(tau_thrust) -> Mixer/4(tau_thrust), Scope11/4, Scope5/1  "stg. 0-1"
  [O_R] -> Selector/1
  Selector/1 -> Switch2/1
  Constant/1 -> Switch2/3
  Selector7/1 -> Switch1/1
  [O_R] -> Selector7/1
  Constant1/1 -> Switch1/3

== system softMBD/FCS/filters ==
  Sensors_data : Inport
  Bus Creator : BusCreator  Inputs=4  OutDataTypeStr=Bus: Sensors_filtered
  Bus Selector : BusSelector  OutputSignals=timestamp_ms,status,axayaz_s,pqr_sf,pressure_s,mxmymz_s,altitude_s,temp_s,vbat_s
  Constant : Constant  Value=g*[0 0 -1]  OutDataTypeStr=single
  Scope{2..7} (6 alike) : Scope
      Scope2 settings: ActiveDisplayYMinimum=-1  ActiveDisplayYMaximum=1  DataLoggingVariableName=ScopeData49
      Scope3 settings: ActiveDisplayYMinimum=-1  ActiveDisplayYMaximum=1  DataLoggingVariableName=ScopeData50
      Scope4 settings: ActiveDisplayYMinimum=-1  ActiveDisplayYMaximum=1  DataLoggingVariableName=ScopeData51
      Scope5 settings: ActiveDisplayYMinimum=-1  ActiveDisplayYMaximum=1  DataLoggingVariableName=ScopeData52
      Scope6 settings: ActiveDisplayYMinimum=-1  ActiveDisplayYMaximum=1  DataLoggingVariableName=ScopeData76
      Scope7 settings: ActiveDisplayYMinimum=-116.31371736526489  ActiveDisplayYMaximum=81.937744617462158  DataLoggingVariableName=ScopeData78
  Subsystem : Subsystem
  Subsystem1 : Subsystem
  Terminator{,1..5} (6 alike) : Terminator
  Transfer Fcn : discretizing/Discretized Transfer Fcn  Numerator=[1]  Denominator=[0.1 1]  AbsTol=auto  SampleTime=0.005  method=zoh  Wc=0
  Transfer Fcn1 : discretizing/Discretized Transfer Fcn  Numerator=[1]  Denominator=[0.1 1]  AbsTol=auto  SampleTime=0.005  method=zoh  Wc=0
  Transfer Fcn2 : discretizing/Discretized Transfer Fcn  Numerator=[1]  Denominator=[0.1 1]  AbsTol=auto  SampleTime=0.005  method=zoh  Wc=0
  pqr_LPF : Subsystem
  pqr_LPF1 : Subsystem
  Sensors_filtered : Outport
  wires:
  Bus Selector/3 -> pqr_LPF1/1(1)  "<axayaz_s>"
  Bus Selector/1 -> Terminator/1  "<timestamp_ms>"
  Bus Selector/2 -> Terminator1/1  "<status>"
  Bus Selector/9 -> Terminator3/1  "<vbat_s>"
  Bus Selector/6 -> Transfer Fcn2/1  "<mxmymz_s>"
  Bus Selector/7 -> Transfer Fcn1/1  "<altitude_s>"
  Bus Selector/8 -> Transfer Fcn/1  "<temp_s>"
  Transfer Fcn1/1 -> Scope7/1, [B]  "pressure_f"
  Bus Selector/5 -> Terminator2/1  "<pressure_s>"
  Bus Selector/4 -> pqr_LPF/1(p,q,r)  "<pqr_sf>"
  pqr_LPF/1(p,q,r_f) -> Scope5/1, Bus Creator/4, Subsystem1/2(p,q,r_f)  "pqr_s"
  Transfer Fcn/1 -> Terminator4/1  "temp_f"
  Transfer Fcn2/1 -> Terminator5/1  "alt_f"
  [B] -> Subsystem/1(pressure_f)  "pressure_f"
  Subsystem/1(x,y,z) -> Scope2/1, Bus Creator/1  "xyz_s"
  Subsystem/2(dx,dy,dz) -> Scope3/1, Bus Creator/2  "dxdydz_s"
  Subsystem1/1(orient_earth) -> Subsystem/3(orient_earth), Scope4/1, Bus Creator/3  "rollpitchyaw_s"
  Bus Creator/1 -> Sensors_filtered/1
  Sensors_data/1 -> Bus Selector/1
  Constant/1 -> ?
  pqr_LPF1/1(ax,ay,az) -> Scope6/1, Subsystem1/1(ax,ay,ax_f), Subsystem/2(ax,ay,ax_f)  "ax,ay,ax_f"

== system softMBD/FCS/value scaling ==
  <orient_ref> : Inport
  Constant : Constant  Value=FPV_mass*g  OutDataTypeStr=single
  Dead Zone : DeadZone  LowerValue=-0.03  UpperValue=0.03
  Demux : Demux
  Gain : Gain  Gain=0.5236  ParamDataTypeStr=single
  Gain1 : Gain  Gain=0.5236  OutDataTypeStr=single
  Gain2 : Gain  Gain=3.49  OutDataTypeStr=single
  Gain3 : Gain  Gain=(FPV_mass*g)-0.5  OutDataTypeStr=single
  Mux : Mux
  Saturation : Saturate  UpperLimit=1  LowerLimit=-1
  Sum : Sum  Inputs=|++
  Out1 : Outport
  wires:
  Mux/1 -> Out1/1
  <orient_ref>/1 -> Saturation/1
  Saturation/1 -> Dead Zone/1
  Demux/2 -> Gain1/1  "pitch"
  Demux/1 -> Gain/1  "roll"
  Demux/3 -> Gain2/1  "yaw"
  Demux/4 -> Gain3/1  "throttle"
  Gain/1 -> Mux/1  "<-0.5236;0.5236> [Rad]"
  Gain1/1 -> Mux/2  "<-0.5236;0.5236> [Rad]"
  Gain2/1 -> Mux/3  "<-3.49;3.49> [Rad/s]"
  Gain3/1 -> Sum/1
  Constant/1 -> Sum/2
  Sum/1 -> Mux/4  "<0.5;9,31> [N]"
  Dead Zone/1 -> Demux/1

== system softMBD/Model/Subsystem ==
  FCS : Inport
  Enviroment : Inport  Port=2
  DCM(angeles) : Inport  Port=3
  V_b : Inport  Port=4
  omega_b : Inport  Port=5
  Add : Sum  Inputs=+++
  Add1 : Sum  Inputs=++++
  Bus Selector : BusSelector  OutputSignals=Gravity_ned,air_density
  Constant : Constant  Value=0
  Constant1 : Constant  Value=0
  Data Type Conversion{1..5} (5 alike) : DataTypeConversion  OutDataTypeStr=double  SaturateOnIntegerOverflow=off  RndMeth=Floor
  Demux : Demux
  Gain{,1..3} (4 alike) : Gain  Gain=6.0/1999
  Manual Switch : ManualSwitch  CurrentSetting=0
  Motor Forces and Torques : Subsystem
  Mux : Mux  Inputs=3
  Saturation : Saturate  UpperLimit=25  LowerLimit=-25  OutDataTypeStr=double
  Scope : Scope  NumInputPorts=3
      settings: ActiveDisplayYMinimum=-0.000142277817061181  ActiveDisplayYMaximum=0.00017675284388450334  DataLoggingVariableName=ScopeData69
  Scope1 : Scope
      settings: ActiveDisplayYMinimum=-1  ActiveDisplayYMaximum=1  DataLoggingVariableName=ScopeData71
  Scope2 : Scope
      settings: ActiveDisplayYMinimum=-1.3749999694671553  ActiveDisplayYMaximum=12.3749997252044  DataLoggingVariableName=ScopeData69
  drag forces : Subsystem
  gravity forces : Subsystem
  F_xyz : Outport
  m_xyz : Outport  Port=2
  wires:
  Add/1 -> Saturation/1
  Bus Selector/1 -> Data Type Conversion1/1  "<Gravity_ned>"
  Enviroment/1 -> Bus Selector/1
  DCM(angeles)/1 -> gravity forces/2(DCM(angeles))
  gravity forces/1(Out1) -> Scope/1, Add/1
  drag forces/1(Out1) -> Add/2, Scope/2
  Bus Selector/2 -> Data Type Conversion3/1  "<air_density>"
  V_b/1 -> Scope1/1, Data Type Conversion2/1
  omega_b/1 -> Data Type Conversion4/1
  FCS/1 -> Data Type Conversion5/1
  Motor Forces and Torques/1(Motor Forces) -> Scope/3, Add/3
  Motor Forces and Torques/2(Motor Torques) -> m_xyz/1
  Saturation/1 -> Manual Switch/1
  Data Type Conversion3/1 -> drag forces/1(pressure), Motor Forces and Torques/2(Density)
  Data Type Conversion1/1 -> gravity forces/1(gravity)
  Data Type Conversion2/1 -> Motor Forces and Torques/1(Vb), drag forces/2(V_b)
  Data Type Conversion4/1 -> Motor Forces and Torques/3(pqr)
  Data Type Conversion5/1 -> Demux/1, Motor Forces and Torques/4(Motor Commands)
  Manual Switch/1 -> Scope2/1, F_xyz/1
  Mux/1 -> Manual Switch/2
  Constant/1 -> Mux/1
  Constant1/1 -> Mux/2
  Demux/1 -> Gain/1
  Demux/2 -> Gain1/1
  Demux/4 -> Gain3/1
  Demux/3 -> Gain2/1
  Gain3/1 -> Add1/4
  Gain2/1 -> Add1/3
  Gain1/1 -> Add1/2
  Gain/1 -> Add1/1
  Add1/1 -> Mux/3

== system softMBD/Sensors/Subsystem ==
  In1 : Inport
  Bus Creator : BusCreator  Inputs=9  OutDataTypeStr=Bus: sensors_mes
  Demux : Demux  Outputs=8
  Mux1 : Mux  Inputs=3
  Mux2 : Mux  Inputs=3
  Subsystem : Subsystem
  Zero{,1..3} (4 alike) : Constant  Value=0  OutDataTypeStr=single
  Out1 : Outport
  wires:
  In1/1 -> Demux/1
  Zero/1 -> Bus Creator/1  "timestamp_ms"
  Zero1/1 -> Bus Creator/2  "status"
  Mux1/1 -> Bus Creator/3  "axayaz_s"
  Mux2/1 -> Bus Creator/4  "pqr_sf"
  Subsystem/1(Out1) -> Bus Creator/5  "mxmymz_s"
  Demux/1 -> Mux1/1
  Demux/2 -> Mux1/2
  Demux/3 -> Mux1/3
  Demux/4 -> Mux2/1
  Demux/5 -> Mux2/2
  Demux/6 -> Mux2/3
  Demux/7 -> Bus Creator/6  "altitude_s"
  Demux/8 -> Bus Creator/7  "pressure_s"
  Zero2/1 -> Bus Creator/8  "temp_s"
  Zero3/1 -> Bus Creator/9  "vbat_s"
  Bus Creator/1 -> Out1/1

== system softMBD/Sensors/Subsystem1 ==
  In1 : Inport
  In2 : Inport  Port=2
  <Accel_b> : Inport  Port=3
  Bus Creator : BusCreator  Inputs=9  OutDataTypeStr=Bus: sensors_mes
  Data Type Conversion1 : DataTypeConversion  OutDataTypeStr=single  SaturateOnIntegerOverflow=off  RndMeth=Floor
  Data Type Conversion2 : DataTypeConversion  OutDataTypeStr=single  SaturateOnIntegerOverflow=off  RndMeth=Floor
  Data Type Conversion3 : DataTypeConversion  OutDataTypeStr=single  SaturateOnIntegerOverflow=off  RndMeth=Floor
  Scope : Scope  NumInputPorts=3
      settings: ActiveDisplayYMinimum=-53.753177344799042  ActiveDisplayYMaximum=12.552743136882782  DataLoggingVariableName=ScopeData49
  Subsystem : Subsystem
  Zero{,1..4} (5 alike) : Constant  Value=0  OutDataTypeStr=single
  Out1 : Outport
  wires:
  Zero/1 -> Bus Creator/1  "timestamp_ms"
  Zero1/1 -> Bus Creator/2  "status"
  Subsystem/1(Out1) -> Bus Creator/5  "mxmymz_s"
  Zero2/1 -> Bus Creator/8  "temp_s"
  Zero3/1 -> Bus Creator/9  "vbat_s"
  Bus Creator/1 -> Out1/1
  Zero4/1 -> Bus Creator/7  "pressure_s"
  Data Type Conversion3/1 -> Scope/3, Bus Creator/6  "altitude_s"
  Data Type Conversion2/1 -> Scope/1, Bus Creator/3  "axayaz_s"
  Data Type Conversion1/1 -> Scope/2, Bus Creator/4  "pqr_sf"
  In1/1 -> Data Type Conversion3/1  "altitude_s"
  In2/1 -> Data Type Conversion1/1  "pqr_sf"
  <Accel_b>/1 -> Data Type Conversion2/1  "axayaz_s"

== system softMBD/FCS/Controller/Mixer ==
  note: wejscie to siła w Newtonach zależna od ciężaru założenie, że 1p newtownów to beziecnzy zapsa więc po 5 na każdy silnik wyjście to steorwaniem przetowrnica w zakresie 48-2047 więc gain 255.875 to przlicznie zakresu 0-8 na 255.875 żebyu mieć zapas i zobacyzmy jak to lata wartości są eksperymenalne , zakłądam 10 bo ejdnye na podsatiwe rówmnoważenia m*g
  tau_roll : Inport
  tau_pitch : Inport  Port=2
  tau_yaw : Inport  Port=3
  tau_thrust : Inport  Port=4
  Bias : Bias  Bias=48  SaturateOnIntegerOverflow=off
  Matrix Multiply : Product  Multiplication=Matrix(*)
  Mux : Mux
  Saturation : Saturate  UpperLimit=4.24  LowerLimit=0.15
  Saturation5 : Saturate  UpperLimit=2047  LowerLimit=48
  ThrustToMotorCommand : Gain  Gain=(2047-48)/4.24  OutDataTypeStr=single
  TorqueTotalThrustToThrustPerMotor : Constant  Value=Q2Ts  OutDataTypeStr=single
  thrusts_refout : Outport
  wires:
  tau_roll/1 -> Mux/4
  tau_pitch/1 -> Mux/3
  tau_yaw/1 -> Mux/2
  tau_thrust/1 -> Mux/1
  TorqueTotalThrustToThrustPerMotor/1 -> Matrix Multiply/1
  Mux/1 -> Matrix Multiply/2
  Saturation/1 -> ThrustToMotorCommand/1
  Matrix Multiply/1 -> Saturation/1
  Saturation5/1 -> thrusts_refout/1
  ThrustToMotorCommand/1 -> Bias/1
  Bias/1 -> Saturation5/1

== system softMBD/FCS/Controller/Thrust_controller ==
  Mode : Inport
  thorttle : Inport  Port=2
  z_s : Inport  Port=3
  dz_s : Inport  Port=4
  AND : Logic  IconShape=distinctive  AllPortsSameDT=off  OutDataTypeStr=boolean
  Abs : Abs  SaturateOnIntegerOverflow=off
  Compare To Constant : simulink/Logic and Bit Operations/Compare To Constant  relop=<=  const=0.5  OutDataTypeStr=boolean
  Constant : Constant  Value=g*FPV_mass*0.97  OutDataTypeStr=single
  Constant2 : Constant  Value=0
  Discrete Derivative : simulink/Discrete/Discrete Derivative  gainval=1.0  ICPrevScaledInput=0.0  OutMin=[]  OutMax=[]  OutDataType=fixdt(1, 16)  OutScaling=2^-10  DoSatur=off
  Gain1 : Gain  OutDataTypeStr=single
  Gain5 : Gain  Gain=3  OutDataTypeStr=single
  Gain6 : Gain  Gain=-1
  Integrator2 : DiscreteIntegrator  gainval=ki_t  ExternalReset=rising  SampleTime=0.005  LimitOutput=on  UpperSaturationLimit=0.5  LowerSaturationLimit=-0.5  ICPrevOutput=DiscIntNeverNeededParam  ICPrevScaledInput=DiscIntNeverNeededParam  mask(DiscretizedDiscreteIntegrator){}
      mask init:
      | %zoh
  NOT : Logic  Operator=NOT  IconShape=distinctive  AllPortsSameDT=off  OutDataTypeStr=boolean
  Rate Limiter : RateLimiter  RisingSlewLimit=20  FallingSlewLimit=-10  SampleTimeMode=inherited
  Rate Limiter1 : RateLimiter  RisingSlewLimit=20  FallingSlewLimit=-10  SampleTimeMode=inherited
  S-R Flip-Flop : simulink_extras/Flip Flops/S-R Flip-Flop  initial_condition=0
  Saturation1 : Saturate  UpperLimit=13.0  LowerLimit=0.5
  Scope : Scope
      settings: ActiveDisplayYMinimum=-116.31371736526489  ActiveDisplayYMaximum=81.937744617462158  DataLoggingVariableName=ScopeData39
  Scope2 : Scope  NumInputPorts=2
      settings: ActiveDisplayYMinimum=-19.214691281318665  ActiveDisplayYMaximum=14.506928563117981  DataLoggingVariableName=ScopeData55
  Scope3 : Scope  NumInputPorts=3
      settings: ActiveDisplayYMinimum=-0.53203654289245583  ActiveDisplayYMaximum=9.7883288860321045  DataLoggingVariableName=ScopeData58
  Sum1 : Sum  Inputs=++|
  Sum3 : Sum  Inputs=+-|
  Sum4 : Sum  Inputs=+|+|+
  Switch : Switch  Criteria=u2 > Threshold  SaturateOnIntegerOverflow=off  InputSameDT=off
  Switch2 : Switch  Criteria=u2 > Threshold  OutDataTypeStr=single  SaturateOnIntegerOverflow=off  InputSameDT=off
  Switch3 : Switch  Criteria=u2 > Threshold  SaturateOnIntegerOverflow=off  InputSameDT=off
  Terminator : Terminator
  Terminator1 : Terminator
  Unit Delay : UnitDelay  SampleTime=-1  HasFrameUpgradeWarning=on
  tau_thrust : Outport
  wires:
  Switch2/1 -> Rate Limiter/1  "wynik"
  Sum1/1 -> Scope3/1, Switch2/1
  z_s/1 -> Switch3/3, Scope/1, Sum3/2, Discrete Derivative/1
  Mode/1 -> NOT/1, AND/2, Switch2/2, Integrator2/2
  Sum3/1 -> Scope2/2, Gain1/1, Gain5/1
  Gain5/1 -> Sum4/2
  Integrator2/1 -> Sum4/3
  Gain6/1 -> Rate Limiter1/1
  Gain1/1 -> Integrator2/1
  Unit Delay/1 -> Switch3/1
  Switch3/1 -> Unit Delay/1, Sum3/1
  Switch/1 -> Sum1/2
  Abs/1 -> Compare To Constant/1
  Sum4/1 -> Scope2/1, Switch/1  "pid"
  Constant2/1 -> Switch/3
  Saturation1/1 -> Scope3/3, tau_thrust/1
  Discrete Derivative/1 -> Gain6/1, Abs/1
  Compare To Constant/1 -> AND/1
  thorttle/1 -> Switch2/3, Scope3/2
  NOT/1 -> S-R Flip-Flop/2
  AND/1 -> S-R Flip-Flop/1
  S-R Flip-Flop/1 -> Switch/2, Switch3/2
  S-R Flip-Flop/2 -> Terminator/1
  Rate Limiter1/1 -> Sum4/1
  dz_s/1 -> Terminator1/1
  Rate Limiter/1 -> Saturation1/1
  Constant/1 -> Sum1/1
